simulink model "NN_v01"  (R2018b)
settings: Solver=VariableStepAuto  StartTime=0.0  StopTime=10.0  RelTol=1e-3
values from neighbouring files (symbols this model uses):
  B = 0.5    [Matlab_Newton_simulation_v01.m]    (also in NewtonMethod.m; NewtonMethod_2.m = 0.3; System_parameters.m = 0.3)
  b = f    (= 0.01)    [Matlab_Newton_simulation_v01.m]    (also in NewtonMethod.m; System_parameters.m)
  in_NN_data = [0 -100 -100 -100 -100 -100 -100 -100 -100 -100 -100 -100 ... (160801 elements, 401x401)]    [NN_IO_data.mat]    (also in NN_generate_input_data.m = con2seq(in_NN_data); NN_modelling_v02.m = con2seq(in_NN_data); NN_modelling_v03.m = con2seq(in_NN_data))
  l = 0.1    [Matlab_Newton_simulation_v01.m]    (also in NewtonMethod.m; NewtonMethod_2.m; System_parameters.m)
  m = 0.04    [Matlab_Newton_simulation_v01.m]    (also in NewtonMethod.m = 0.1; NewtonMethod_2.m; System_parameters.m)
  R = 1    [Matlab_Newton_simulation_v01.m]    (also in NewtonMethod.m; NewtonMethod_2.m = 0.1; System_parameters.m = 0.1)
libraries: neural x128
(part 4 of 5)

== system NN_v01/NARX Neural Network/Layer 2/Delays 1 ==
  "p{2}" : Inport  PortDimensions=10  SampleTime=1
      mask Display: e = 0.06;c1 = [120 230 180]/255;c2 = ([120 230 180]+0)/(256+128);c3 = ([120 230 180]+128)/(256+128);patch([0 1 1 0],[0 0 1 1],c1);patch([0 1 1 1-e 1-e 0+e],[0 0 1 1-e 0+e 0+e],c2);patch([0 0 1 1-e 0+e 0+e],[0 1 1 1-e 1-e 0+e],c3);plot([0 1 1 0 0],[0 0 1 1 0]);
  mux : Mux  Inputs=1
      mask Display: e = 0.06;c1 = [120 150 230]/255;c2 = ([120 150 230]+0)/383;c3 = ([120 150 230]+128)/383;patch([0 1 1 0],[0 0 1 1],c1);patch([0 1 1 1-e 1-e 0+e],[0 0 1 1-e 0+e 0+e],c2);patch([0 0 1 1-e 0+e 0+e],[0 1 1 1-e 1-e 0+e],c3);plot([0 1 1 0 0],[0 0 1 1 0]);disp('Mux')
  "pd{2,1}" : Outport
      mask Display: e = 0.06;c1 = [120 230 180]/255;c2 = ([120 230 180]+0)/(256+128);c3 = ([120 230 180]+128)/(256+128);patch([0 1 1 0],[0 0 1 1],c1);patch([0 1 1 1-e 1-e 0+e],[0 0 1 1-e 0+e 0+e],c2);patch([0 0 1 1-e 0+e 0+e],[0 1 1 1-e 1-e 0+e],c3);plot([0 1 1 0 0],[0 0 1 1 0]);
  wires:
  "p{2}"/1 -> mux/1
  mux/1 -> "pd{2,1}"/1
